simulink model "system_sim"  (R2015a)
settings: Solver=ode45  StartTime=0.0  StopTime=10.0  RelTol=1e-3
libraries: simulink x1
settings Model: Creator=marco  LastModifiedBy=mrclpt

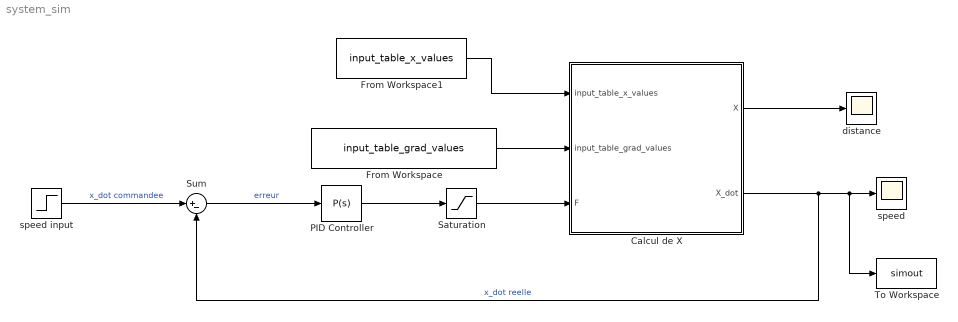
== system system_sim ==
  Calcul de X : Subsystem
  From Workspace : FromWorkspace  VariableName=input_table_grad_values  SampleTime=0
  From Workspace1 : FromWorkspace  VariableName=input_table_x_values  SampleTime=0
  PID Controller : simulink/Continuous/PID Controller  Controller=P  TimeDomain=Continuous-time  SampleTime=-1  IntegratorMethod=Forward Euler  FilterMethod=Forward Euler  Form=Parallel  UseFilter=on  ControllerParametersSource=internal  P=1  I=0  D=0  N=100  InitialConditionSource=internal  InitialConditionForIntegrator=0  InitialConditionForFilter=0  ExternalReset=none  LimitOutput=off  UpperSaturationLimit=inf  LowerSaturationLimit=-inf  LinearizeAsGain=on  AntiWindupMode=none  Kb=1  TrackingMode=off  Kt=1  PParamMin=[]  PParamMax=[]  IParamMin=[]  IParamMax=[]  DParamMin=[]  DParamMax=[]  NParamMin=[]  NParamMax=[]  KbParamMin=[]  KbParamMax=[]  KtParamMin=[]  KtParamMax=[]  POutMin=[]  POutMax=[]  IOutMin=[]  IOutMax=[]  DOutMin=[]  DOutMax=[]  NOutMin=[]  NOutMax=[]  KbOutMin=[]  KbOutMax=[]  KtOutMin=[]  KtOutMax=[]  IntegratorOutMin=[]  IntegratorOutMax=[]  FilterOutMin=[]  FilterOutMax=[]  SumOutMin=[]  SumOutMax=[]  SumI1OutMin=[]  SumI1OutMax=[]  SumI2OutMin=[]  SumI2OutMax=[]  SumI3OutMin=[]  SumI3OutMax=[]  SumDOutMin=[]  SumDOutMax=[]  SaturationOutMin=[]  SaturationOutMax=[]  IntegratorContinuousStateAttributes=''  IntegratorStateMustResolveToSignalObject=off  IntegratorRTWStateStorageClass=Auto  FilterContinuousStateAttributes=''  FilterStateMustResolveToSignalObject=off  FilterRTWStateStorageClass=Auto  DifferentiatorICPrevScaledInput=0  DifferentiatorOutMin=[]  DifferentiatorOutMax=[]
  Saturation : Saturate  UpperLimit=150  LowerLimit=-150
  Sum : Sum  Inputs=|+-
  To Workspace : ToWorkspace  VariableName=simout  SampleTime=-1
      settings: Save2DSignal=2-D array (concatenate along first dimension)
  distance : Scope
  speed : Scope
  speed input : Step  Time=0  After=4.16  SampleTime=1
  wires:
  PID Controller/1 -> Saturation/1
  Sum/1 -> PID Controller/1  "erreur"
  Calcul de X/2(X_dot) -> To Workspace/1, speed/1, Sum/2  "x_dot reelle"
  Calcul de X/1(X) -> distance/1
  speed input/1 -> Sum/1  "x_dot commandee"
  Saturation/1 -> Calcul de X/3(F)
  From Workspace1/1 -> Calcul de X/1(input_table_x_values)
  From Workspace/1 -> Calcul de X/2(input_table_grad_values)

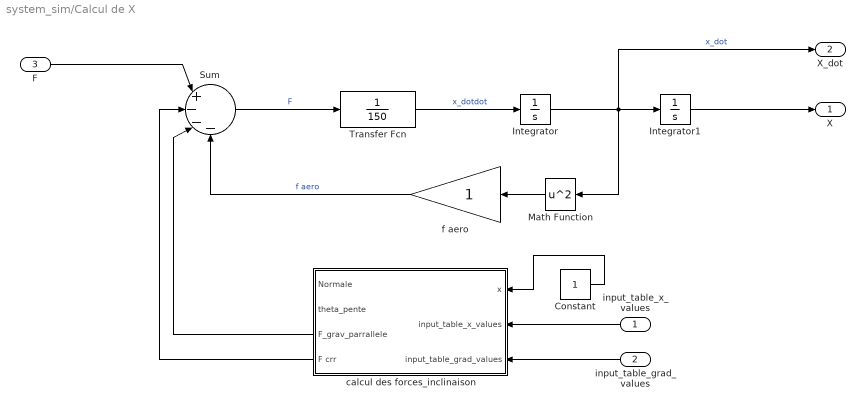
== system system_sim/Calcul de X ==
  input_table_x_values : Inport
  input_table_grad_values : Inport  Port=2
  F : Inport  Port=3
  Constant : Constant
  Integrator : Integrator
  Integrator1 : Integrator
  Math Function : Math  Operator=square  SaturateOnIntegerOverflow=on
  Sum : Sum  Inputs=|+---
  Transfer Fcn : TransferFcn  Denominator=[150]
  calcul des forces_inclinaison : Subsystem
  f aero : Gain
  X : Outport
  X_dot : Outport  Port=2
  wires:
  Sum/1 -> Transfer Fcn/1  "F"
  Transfer Fcn/1 -> Integrator/1  "x_dotdot"
  Integrator/1 -> Math Function/1, X_dot/1, Integrator1/1  "x_dot"
  f aero/1 -> Sum/4  "f aero"
  F/1 -> Sum/1
  Integrator1/1 -> X/1
  calcul des forces_inclinaison/3(F_grav_parrallele) -> Sum/3
  calcul des forces_inclinaison/4(F crr) -> Sum/2
  Math Function/1 -> f aero/1
  input_table_x_values/1 -> calcul des forces_inclinaison/2(input_table_x_values)
  input_table_grad_values/1 -> calcul des forces_inclinaison/3(input_table_grad_values)
  Constant/1 -> calcul des forces_inclinaison/1(x)

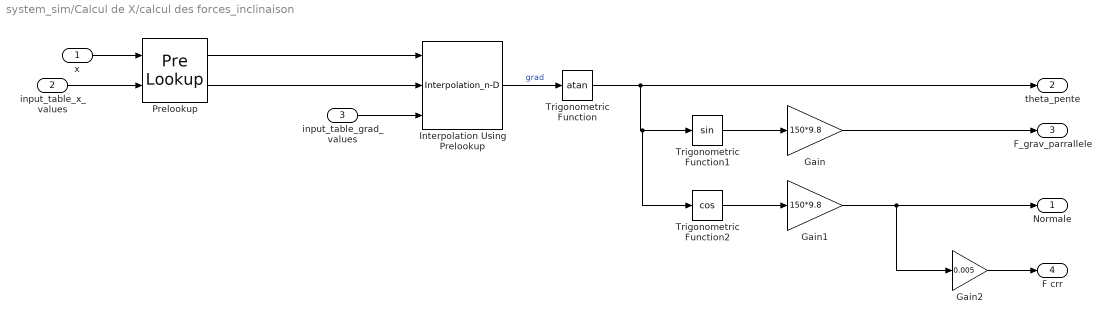
== system system_sim/Calcul de X/calcul des forces_inclinaison ==
  x : Inport
  input_table_x_values : Inport  Port=2
  input_table_grad_values : Inport  Port=3
  Gain : Gain  Gain=150*9.8
  Gain1 : Gain  Gain=150*9.8
  Gain2 : Gain  Gain=0.005
  Interpolation Using Prelookup : Interpolation_n-D  NumberOfTableDimensions=1  TableSource=Input port  InternalRulePriority=Speed
      settings: InputPortMap=u0,u1,p2
  Prelookup : PreLookup  BreakpointsDataSource=Input port  BreakpointsData=[10:10:110]  ExtrapMethod=Linear
      settings: InputPortMap=u0,p1
  Trigonometric Function : Trigonometry  Operator=atan
  Trigonometric Function1 : Trigonometry
  Trigonometric Function2 : Trigonometry  Operator=cos
  Normale : Outport
  theta_pente : Outport  Port=2
  F_grav_parrallele : Outport  Port=3
  F crr : Outport  Port=4
  wires:
  x/1 -> Prelookup/1
  Interpolation Using Prelookup/1 -> Trigonometric Function/1  "grad"
  Trigonometric Function/1 -> Trigonometric Function2/1, Trigonometric Function1/1, theta_pente/1
  Trigonometric Function1/1 -> Gain/1
  Trigonometric Function2/1 -> Gain1/1
  Gain1/1 -> Gain2/1, Normale/1
  Gain/1 -> F_grav_parrallele/1
  Gain2/1 -> F crr/1
  Prelookup/1 -> Interpolation Using Prelookup/1
  Prelookup/2 -> Interpolation Using Prelookup/2
  input_table_grad_values/1 -> Interpolation Using Prelookup/3
  input_table_x_values/1 -> Prelookup/2
